simulink model "sim13_constantes"  (R2015b)
settings: Solver=VariableStepAuto  StartTime=0.0  StopTime=20.0  RelTol=1e-3
values from neighbouring files (symbols this model uses):
  dy_inicial = 0    [Lab2.m]
  k1 = 1/yl    (= 10)    [Lab2.m]    (also in u_valor.m = 1/yl)
  k2 = sqrt(2*k1)    [Lab2.m]    (also in u_valor.m)
  y_inicial = 1    [Lab2.m]
  yl = 0.1    [Lab2.m]
undefined symbols (not defined in the file or in its folder): sigbuilder_block
settings Model: Creator=Alice  LastModifiedBy=Alice

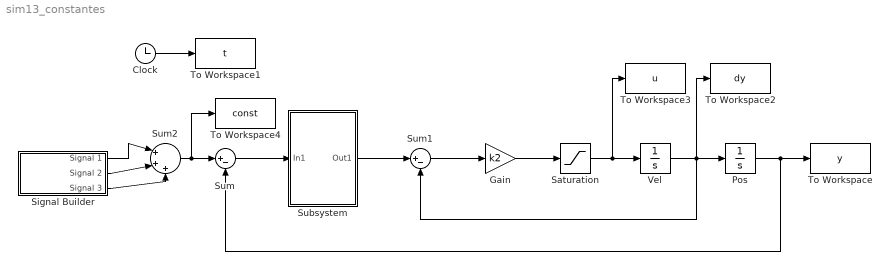
== system sim13_constantes ==
  Clock : Clock
  Gain : Gain  Gain=k2
  Pos : Integrator  InitialCondition=y_inicial
  Saturation : Saturate  UpperLimit=1  LowerLimit=-1
  Signal Builder : Subsystem  Tag=STV Subsys  LoadFcn=sigbuilder_block('load');  StartFcn=sigbuilder_block('start');  StopFcn=sigbuilder_block('stop');  ClipboardFcn=sigbuilder_block('clipboard');  mask(Sigbuilder block){}
      mask help: Simulink:masks:SigbuilderBlock_MD
      mask init:
      | if ~strcmp(get_param(bdroot(gcbh),'SimulationStatus'),'stopped') tuvar = sigbuilder_block('maskInit'); end
      settings: CopyFcn=sigbuilder_block('copy');  DeleteFcn=sigbuilder_block('delete');  ModelCloseFcn=sigbuilder_block('modelClose');  PreSaveFcn=sigbuilder_block('preSave');  PauseFcn=sigbuilder_block('pause');  ContinueFcn=sigbuilder_block('continue');  NameChangeFcn=sigbuilder_block('namechange');  OpenFcn=sigbuilder_block('open',[0 30 1024.5 488.25 ]);  CloseFcn=sigbuilder_block('close');
      mask Display: plot(0, 0, 100, 100,[2, 2, 32, 32, 2], [68, 8, 8, 68, 68],[32, 2], [38, 38], [32, 19, 2],[53, 60, 44], [32, 17, 17, 2],[16, 16, 31, 31]);txt = getActiveGroup(gcbh);text(2, 100, txt,'verticalAlignment', 'top');
  Subsystem : Subsystem
  Sum : Sum  Inputs=|+-
  Sum1 : Sum  Inputs=|+-
  Sum2 : Sum  Inputs=|+++
  To Workspace : ToWorkspace  VariableName=y  SampleTime=0.1
  To Workspace1 : ToWorkspace  VariableName=t  SampleTime=0.1
  To Workspace2 : ToWorkspace  VariableName=dy  SampleTime=0.1
  To Workspace3 : ToWorkspace  VariableName=u  SampleTime=0.1
  To Workspace4 : ToWorkspace  VariableName=const  SampleTime=-1
  Vel : Integrator  InitialCondition=dy_inicial
  wires:
  Sum/1 -> Subsystem/1(In1)
  Subsystem/1(Out1) -> Sum1/1
  Sum1/1 -> Gain/1
  Gain/1 -> Saturation/1
  Saturation/1 -> To Workspace3/1, Vel/1
  Vel/1 -> To Workspace2/1, Sum1/2, Pos/1
  Pos/1 -> To Workspace/1, Sum/2
  Clock/1 -> To Workspace1/1
  Sum2/1 -> To Workspace4/1, Sum/1
  Signal Builder/1(Signal 1) -> Sum2/1
  Signal Builder/2(Signal 2) -> Sum2/2
  Signal Builder/3(Signal 3) -> Sum2/3

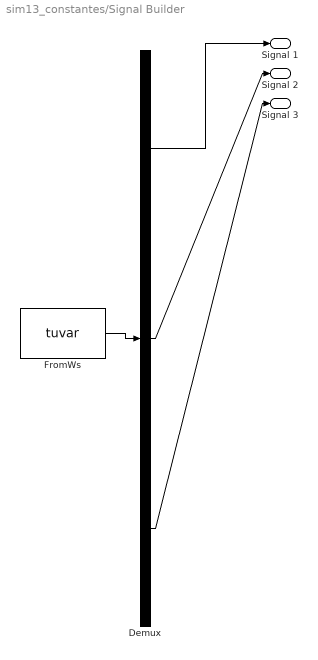
== system sim13_constantes/Signal Builder ==
  Demux : Demux  Tag=STV Demux  Outputs=3
  FromWs : FromWorkspace  Tag=STV FromWs  VariableName=tuvar  SampleTime=0
      SigBuilderData=|
      | common.afterFinalStr = 'Extrapolate'
      | common.sampleTime = 0
      | dataSet.timeRange = [0 20]
      | dataSet.name = 'Group 1'
      | sbobj.Groups.Name = 'Group 1'
      | sbobj.Groups.Signals(1).Name = 'Signal 1'
      | sbobj.Groups.Signals(1).XData = [0 5 5 20]
      | sbobj.Groups.Signals(1).YData = [0 0 1 1]
      | sbobj.Groups.Signals(2).Name = 'Signal 2'
      | sbobj.Groups.Signals(2).XData = [0 10 10 20]
      | sbobj.Groups.Signals(2).YData = [0 0 2 2]
      | sbobj.Groups.Signals(3).Name = 'Signal 3'
      | sbobj.Groups.Signals(3).XData = [0 15 15 20]
      | sbobj.Groups.Signals(3).YData = [0 0 -1 -1]
      | sbobj.Groups.TimeRange = [0 20]
  Signal 1 : Outport  Tag=STV Outport
  Signal 2 : Outport  Tag=STV Outport  Port=2
  Signal 3 : Outport  Tag=STV Outport  Port=3
  wires:
  Demux/1 -> Signal 1/1
  FromWs/1 -> Demux/1
  Demux/2 -> Signal 2/1
  Demux/3 -> Signal 3/1

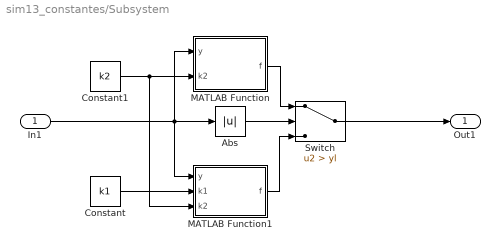
== system sim13_constantes/Subsystem ==
  In1 : Inport
  Abs : Abs
  Constant : Constant  Value=k1
  Constant1 : Constant  Value=k2
  MATLAB Function : MATLAB Function  TreatAsAtomicUnit=on
  MATLAB Function1 : MATLAB Function  TreatAsAtomicUnit=on
  Switch : Switch  Criteria=u2 > Threshold  Threshold=yl
  Out1 : Outport
  wires:
  In1/1 -> Abs/1, MATLAB Function/1(y), MATLAB Function1/1(y)
  Switch/1 -> Out1/1
  MATLAB Function/1(f) -> Switch/1
  Constant/1 -> MATLAB Function1/2(k1)
  MATLAB Function1/1(f) -> Switch/3
  Abs/1 -> Switch/2
  Constant1/1 -> MATLAB Function1/3(k2), MATLAB Function/2(k2)

== matlab function sim13_constantes/Subsystem/MATLAB Function1 ==
  data: y input; k1 input; f output; k2 input
function f = fcn(y,k1,k2)

f=(k1/k2)*(y);

end

== matlab function sim13_constantes/Subsystem/MATLAB Function ==
  data: y input; f output; k2 input
function f = fcn(y,k2)

f=sign(y)*(sqrt(2*abs(y))-(1/k2));

end
